simulink model "getDataIMU6050"  (R2020a)
settings: Solver=VariableStepAuto  StartTime=0.0  StopTime=60  FixedStep=0.005  RelTol=1e-3
undefined symbols (not defined in the file or in its folder): CR, LF, serial
libraries: instrumentlib x2
settings Model: Creator=dangh  LastModifiedBy=dangh

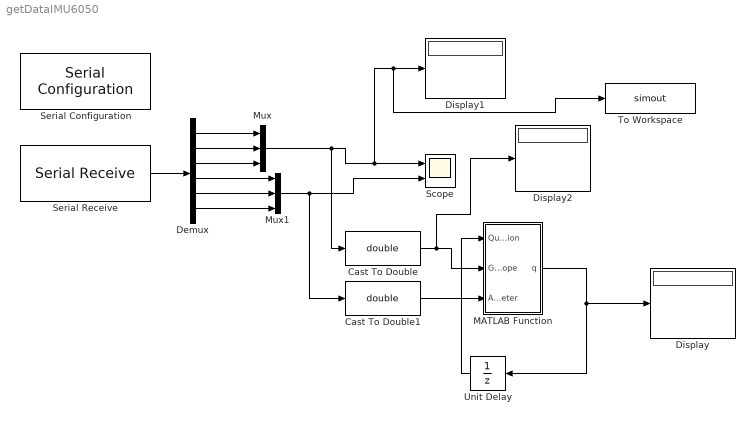
== system getDataIMU6050 ==
  Cast To Double : DataTypeConversion  OutDataTypeStr=double
  Cast To Double1 : DataTypeConversion  OutDataTypeStr=double
  Demux : Demux  Outputs=6
  Display : Display
  Display1 : Display
  Display2 : Display
  MATLAB Function : MATLAB Function  TreatAsAtomicUnit=on
  Mux : Mux  Inputs=3
  Mux1 : Mux  Inputs=3
  Scope : Scope  NumInputPorts=2
  Serial Configuration : instrumentlib/Serial Configuration  Priority=-200000  ComPortMenu=COM8  ComPort=COM8  ObjConstructor=serial('COM8');  BaudRate=115200  DataBits=8  Parity=none  StopBits=1  FlowControl=none  Timeout=10  ByteOrder=LittleEndian
  Serial Receive : instrumentlib/Serial Receive  ComPortMenu=COM8  ComPort=COM8  ObjConstructor=serial('COM8');  Terminator=CR/LF ('\r\n')  DataSize=6  DataType=single  EnableBlockingMode=on  ActionDataUnavailable=Output last received value  CustomValue=0  SampleTime=0.005
  To Workspace : ToWorkspace  VariableName=simout  SampleTime=-1
  Unit Delay : UnitDelay  InitialCondition=[1 0 0 0]  SampleTime=-1  HasFrameUpgradeWarning=on
  wires:
  Serial Receive/1 -> Demux/1
  Demux/1 -> Mux/1
  Demux/2 -> Mux/2
  Demux/3 -> Mux/3
  Demux/4 -> Mux1/1
  Demux/5 -> Mux1/2
  Demux/6 -> Mux1/3
  Mux/1 -> Cast To Double/1, To Workspace/1, Display1/1, Scope/1
  Mux1/1 -> Cast To Double1/1, Scope/2
  MATLAB Function/1(q) -> Unit Delay/1, Display/1
  Cast To Double/1 -> Display2/1, MATLAB Function/2(Gyroscope)
  Cast To Double1/1 -> MATLAB Function/3(Accelerometer)
  Unit Delay/1 -> MATLAB Function/1(Quaternion)

== matlab function getDataIMU6050/MATLAB Function ==
  data: Quaternion input; q output; Gyroscope input; Accelerometer input
%function [residual, xhatOut] = EXTKALMAN(meas, deltat)
function q  = UpdateIMU(Quaternion, Gyroscope, Accelerometer)

% Initialization
SamplePeriod = 1/200;       %5ms
%Quaternion = [1 0 0 0];     % output quaternion describing the Earth relative to the sensor
Beta = 0.1;               	% algorithm gain

     %q = zeros(1,4);
            q = [1 0 0 0]; %Quaternion; % short name local variable for readability

            % Normalise accelerometer measurement
            if(norm(Accelerometer) == 0), return; end	% handle NaN
            Accelerometer = Accelerometer / norm(Accelerometer);	% normalise magnitude

            % Gradient decent algorithm corrective step
            F = [2*(q(2)*q(4) - q(1)*q(3)) - Accelerometer(1)
                2*(q(1)*q(2) + q(3)*q(4)) - Accelerometer(2)
                2*(0.5 - q(2)^2 - q(3)^2) - Accelerometer(3)];
            J = [-2*q(3),	2*q(4),    -2*q(1),	2*q(2)
                2*q(2),     2*q(1),     2*q(4),	2*q(3)
                0,         -4*q(2),    -4*q(3),	0    ];
            step = (J'*F);
            step = step / norm(step);	% normalise step magnitude

            % Compute rate of change of quaternion
            qDot = 0.5 * quaternProd(q, [0 Gyroscope(1) Gyroscope(2) Gyroscope(3)]) - Beta * step';

            % Integrate to yield quaternion
            q = q + qDot * SamplePeriod;
            %Quaternion = q / norm(q); % normalise quaternion
            q = q / norm(q); % normalise quaternion
end
function ab = quaternProd(a, b)
%QUATERNPROD Calculates the quaternion product
%
%   ab = quaternProd(a, b)
%
%   Calculates the quaternion product of quaternion a and b.
%
%   For more information see:
%   http://www.x-io.co.uk/node/8#quaternions
%
%	Date          Author          Notes
%	27/09/2011    SOH Madgwick    Initial release
    ab = zeros(1,4,'double');
    ab(:,1) = a(:,1).*b(:,1)-a(:,2).*b(:,2)-a(:,3).*b(:,3)-a(:,4).*b(:,4);
    ab(:,2) = a(:,1).*b(:,2)+a(:,2).*b(:,1)+a(:,3).*b(:,4)-a(:,4).*b(:,3);
    ab(:,3) = a(:,1).*b(:,3)-a(:,2).*b(:,4)+a(:,3).*b(:,1)+a(:,4).*b(:,2);
    ab(:,4) = a(:,1).*b(:,4)+a(:,2).*b(:,3)-a(:,3).*b(:,2)+a(:,4).*b(:,1);
end
